simulink model "GFLIB_VLog10_BAM_FLT"  (Simulink 8.3)
settings: Solver=ode45  StartTime=0.0  StopTime=10.0  RelTol=1e-3
settings Model: Creator=B37097  LastModifiedBy=B37097
settings DataIOCC: SignalLoggingSaveFormat=Dataset
settings DebuggingCC: UnderspecifiedInitializationDetection=Simplified  StateNameClashWarn=none
settings GRTTargetCC: CombineOutputUpdateFcns=on  GRTInterface=off

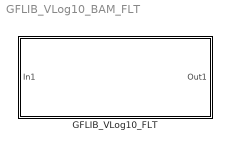
== system GFLIB_VLog10_BAM_FLT ==
  GFLIB_VLog10_FLT : Subsystem  mask(GFLIB_VLog10_FLT){N=32}
      mask prompts: N "Vector length"
      mask help:
      | Bit accurate model of GFLIB_VLog10 function, which computes fast base-10 logarithm of a vector.
      |
      | Note: The vector length parameter N must be <= 4096.
      mask Display:
      | color('black');
      | port_label('input',1,'fltIn');
      | port_label('output',1,'fltOut');
      | color('black');
      | disp('GFLIB_VLog10_FLT');

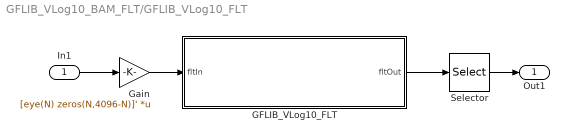
== system GFLIB_VLog10_BAM_FLT/GFLIB_VLog10_FLT ==
  In1 : Inport
  GFLIB_VLog10_FLT : Subsystem  mask(GFLIB_VLog10_FLT){u32N=N}
      mask help: Bit accurate model of GFLIB_VLog10 function, which computes fast base-10 logarithm of a vector.
      mask init:
      | pos = get_param(gcb, 'Position');
      | width = pos(3) - pos(1); 
      | height = pos(4) - pos(2);
      | tX=width/2;tY=height*0.9;
      mask Display: color('black');port_label('input',1,'fltIn');port_label('output',1,'fltOut');color('black');disp('GFLIB_VLog10_FLT');color('blue');text(tX,tY, 'BAM', 'horizontalAlignment', 'center');
  Gain : Gain  Gain=[eye(N) zeros(N,4096-N)]'  Multiplication=Matrix(K*u)
  Selector : Selector  IndexOptions=Starting index (dialog)  OutputSizes=N
  Out1 : Outport
  wires:
  GFLIB_VLog10_FLT/1(fltOut) -> Selector/1
  Gain/1 -> GFLIB_VLog10_FLT/1(fltIn)
  Selector/1 -> Out1/1
  In1/1 -> Gain/1

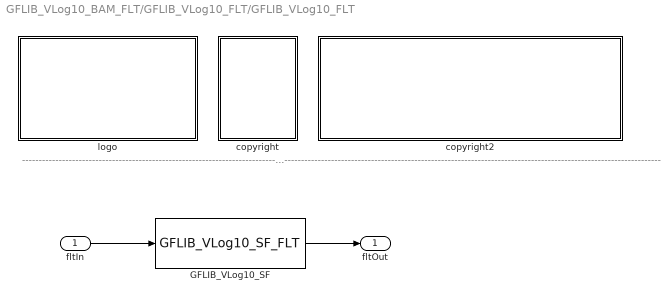
== system GFLIB_VLog10_BAM_FLT/GFLIB_VLog10_FLT/GFLIB_VLog10_FLT ==
  note: ---------------------------------------------------------------------------------------------------------------------------------------------------------------------------------------------------
  fltIn : Inport
  GFLIB_VLog10_SF : S-Function  FunctionName=GFLIB_VLog10_SF_FLT  Parameters=u32N  EnableBusSupport=off
  copyright : Subsystem
      mask Display: text(10,90,'FILE:');text(10,75,'DESRIPTION:');text(10,60,'COPYRIGHT:');text(10,45,'VERSION:');text(10,30,'DATE:')
  copyright2 : Subsystem
      mask Display: text(10,90,'GFLIB_VLog10_BAM_FLT.mdl');text(10,75,'Vector fast base-10 logarithm');text(10,60,'NXP');text(10,45,'1.0');text(10,30,'20-Feb-2017');
  logo : Subsystem
      mask Display: image(imread('logo.jpg'))
  fltOut : Outport
  wires:
  fltIn/1 -> GFLIB_VLog10_SF/1
  GFLIB_VLog10_SF/1 -> fltOut/1

== system GFLIB_VLog10_BAM_FLT/GFLIB_VLog10_FLT/GFLIB_VLog10_FLT/copyright ==

== system GFLIB_VLog10_BAM_FLT/GFLIB_VLog10_FLT/GFLIB_VLog10_FLT/copyright2 ==

== system GFLIB_VLog10_BAM_FLT/GFLIB_VLog10_FLT/GFLIB_VLog10_FLT/logo ==
